simulink model "findDotPositions_th"  (R2018b)
settings: Solver=VariableStepAuto  StartTime=0.0  StopTime=10.0  RelTol=1e-3
libraries: findDotPositions_ul x3
settings Model: Creator=MAE-NCSUCORE  LastModifiedBy=MAE-NCSUCORE

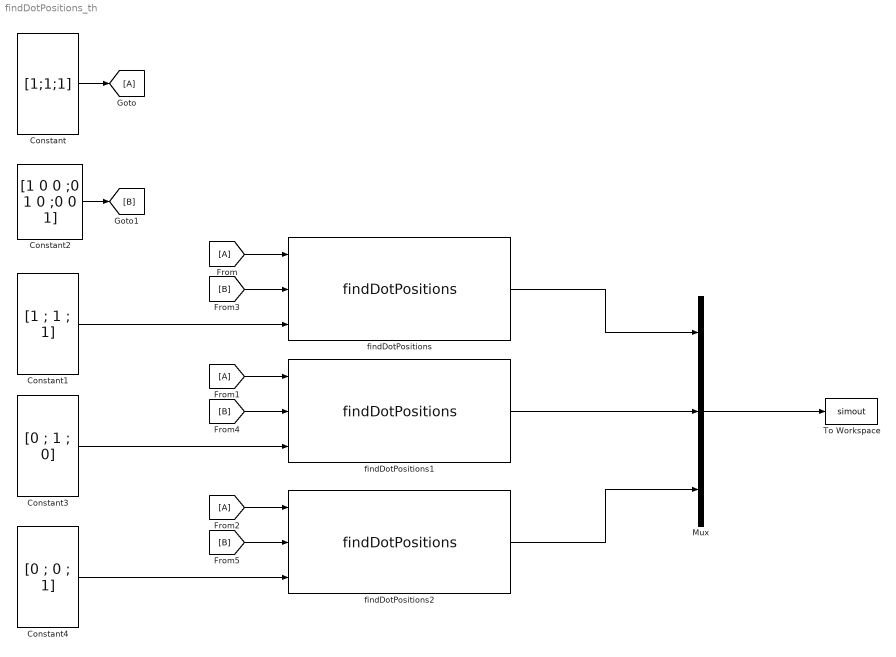
== system findDotPositions_th ==
  Constant : Constant  Value=[1;1;1]
  Constant1 : Constant  Value=[1 ; 1 ; 1]
  Constant2 : Constant  Value=[1 0 0 ;0 1 0 ;0 0 1]
  Constant3 : Constant  Value=[0 ; 1 ; 0]
  Constant4 : Constant  Value=[0 ; 0 ; 1]
  Mux : Mux  Inputs=3
  To Workspace : ToWorkspace  VariableName=simout  SaveFormat=Timeseries  SampleTime=-1
  findDotPositions : findDotPositions_ul/findDotPositions  SystemSampleTime=-1
  findDotPositions1 : findDotPositions_ul/findDotPositions  SystemSampleTime=-1
  findDotPositions2 : findDotPositions_ul/findDotPositions  SystemSampleTime=-1
  wires:
  Constant/1 -> [A]
  Constant2/1 -> [B]
  Constant3/1 -> findDotPositions1/3
  Constant4/1 -> findDotPositions2/3
  Constant1/1 -> findDotPositions/3
  [A] -> findDotPositions/1
  [A] -> findDotPositions2/1
  [A] -> findDotPositions1/1
  [B] -> findDotPositions/2
  [B] -> findDotPositions1/2
  [B] -> findDotPositions2/2
  findDotPositions1/1 -> Mux/2
  findDotPositions2/1 -> Mux/3
  findDotPositions/1 -> Mux/1
  Mux/1 -> To Workspace/1
